simulink model "drone_modelisation_2023aver"  (R2023a)
settings: Solver=VariableStepAuto  StartTime=0.0  StopTime=300  RelTol=1e-3
libraries: sim3dlib x5, matrix_library x3
settings Model: Creator=astro  LastModifiedBy=raphb
settings RTWCC: GPUComputeCapability=5.0

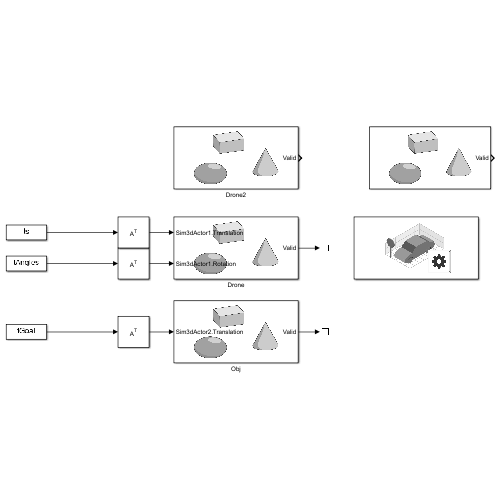
[thumbnail: Simulink's stored preview of the top-level diagram]
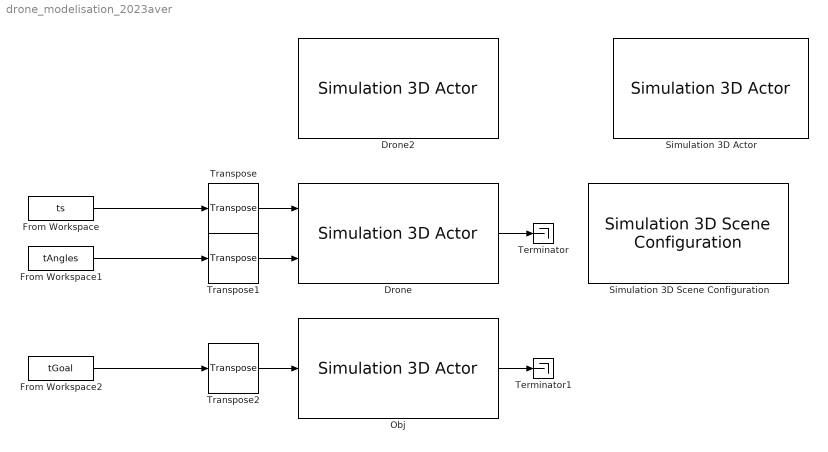
== system drone_modelisation_2023aver ==
  Drone : sim3dlib/Simulation 3D Actor  Priority=1  ActorName=Sim3dActor1  ParentName=Scene Origin  Operation=Create at setup  InitScriptText=|  SampleTime=-1  Translation=single([0 0 1])  Rotation=single([0 0 0])  Scale=single([1 1 1]*.05)  InputsText=Sim3dActor1.Translation Sim3dActor1.Rotation  aMode=5  ActorTag=Sim3dActor1  ActorType=Sim3dActor  ID=1
      | % Reserved keywords:
      | % - Actor : handle to this actor object
      | % - World : handle to the world object
      | 
      | % Examples:
      | 
      | % Create a primitive geometry (optional)
      | Actor.load("Drone Blender fusionner.x3d")
      | World.add(Actor)
  Drone2 : sim3dlib/Simulation 3D Actor  Priority=1  ActorName=Sim3dActor10  ParentName=Scene Origin  Operation=Create at setup  InitScriptText=|  SampleTime=-1  Translation=single([19 9 -0.1])  Rotation=single([0 0 0])  Scale=single([1 1 1])*.1  aMode=5  ActorTag=Sim3dActor10  ActorType=Sim3dActor  ID=10
      | % Reserved keywords:
      | % - Actor : handle to this actor object
      | % - World : handle to the world object
      | 
      | % Examples:
      | 
      | % Create a primitive geometry (optional)
      | Actor.load("Environnement avec couleurs fusionner.x3d")
      | %Actor.load("Les_cubes_moche_environnement.x3d")
      | World.add(Actor)
  From Workspace : FromWorkspace  VariableName=ts  SampleTime=-1
  From Workspace1 : FromWorkspace  VariableName=tAngles
  From Workspace2 : FromWorkspace  VariableName=tGoal
  Obj : sim3dlib/Simulation 3D Actor  Priority=1  ActorName=Sim3dActor2  ParentName=Scene Origin  Operation=Create at setup  InitScriptText=|  SampleTime=-1  Translation=single([0 0 1])  Rotation=single([0 0 0])  Scale=single([1 1 1]*.05)  InputsText=Sim3dActor2.Translation  aMode=5  ActorTag=Sim3dActor2  ActorType=Sim3dActor  ID=2
      | % Reserved keywords:
      | % - Actor : handle to this actor object
      | % - World : handle to the world object
      | 
      | % Examples:
      | 
      | % Create a primitive geometry (optional)
      | Actor.load("Cible fusionner.x3d")
      | World.add(Actor)
  Simulation 3D Actor : sim3dlib/Simulation 3D Actor  ActorName=Sim3dActor11  ParentName=Scene Origin  Operation=Create at setup  InitScriptText=|  SampleTime=-1  Translation=single([14 14 -.2])  Rotation=single([0 0 0])  Scale=single([1 1 1])  aMode=5  ActorTag=Sim3dActor11  ActorType=Sim3dActor  ID=11
      | %Actor.createShape("box", [26.46 26.46 .2]);
      | %Actor.Color = "red";
      | %World.add(Actor)
      settings: LibrarySourceBlock=sl3dlib/Simulation 3D/Simulation 3D Actor
  Simulation 3D Scene Configuration : sim3dlib/Simulation 3D Scene Configuration  Priority=0  ProjectFormat=Default Scenes  SceneDesc=Empty scene  ProjectName=C:\Program Files\MATLAB\R2023a\toolbox\shared\sim3d_projects\automotive_project\UE4\WindowsNoEditor\VehicleSimulation.exe  ScenePath=/Game/Maps/HwStrght  EnableOpenDRIVE=off  vehTagList={'Scene Origin'}  vehTag=Scene Origin  OpVisEn=off  Ts=.02  EnableWindow=on  EnableRemoteAccess=off  EnableWeather=off  SunAltitude=40.0  SunAzimuth=90  clouds=10  wind=1  fog=0  rain=0  EnableGeospatial=off  OriginHeight=200  OriginLatitude=40.744652  OriginLongitude=-73.988864  MapStyle=Aerial  AdditionalAssetIDs=[]  UseAdvancedSunSky=off  SolarTime=11  TimeZone=-5  Day=21  Month=9  Year=2022  UseDaylightSavingTime=on  DSTStartDay=10  DSTStartMonth=3  DSTEndDay=3  DSTEndMonth=11  DSTSwitchHour=2  sensorTag=MainCamera1  sensorId=1  sensorName=MainCamera1  mountLoc=Origin  offsetFlag=off  tmountOffset=[0, 0, 0]  rmountOffset=[0, 0, 0]  HorizontalResolution=1280  VerticalResolution=720  HorizontalFOV=60  mountPoint=[0 0 0]  mountOrientation=[0 0 0]  aMode=5  ID=1  GeoTrigger=Inactive
      settings: LibrarySourceBlock=sl3dlib/Simulation 3D/Environment/Simulation 3D Scene Configuration
  Terminator : Terminator
  Terminator1 : Terminator
  Transpose : matrix_library/Transpose
  Transpose1 : matrix_library/Transpose
  Transpose2 : matrix_library/Transpose
  wires:
  Drone/1 -> Terminator/1
  From Workspace/1 -> Transpose/1
  Transpose/1 -> Drone/1
  From Workspace1/1 -> Transpose1/1
  Transpose1/1 -> Drone/2
  From Workspace2/1 -> Transpose2/1
  Obj/1 -> Terminator1/1
  Transpose2/1 -> Obj/1
